simulink library "FAM_simple_lab_scale"  (R2023b)
settings: Solver=VariableStepAuto  StartTime=0.0  StopTime=10.0  RelTol=1e-3
undefined symbols (not defined in the file): FAM_elasticity, FAM_unstretched_length, FAM_unstretched_radius, FAM_wall_thickness, fiber_angle_alpha
settings Model: Creator=Carson  LastModifiedBy=Carson

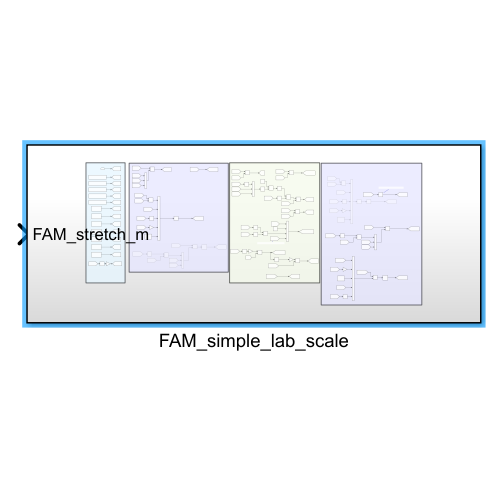
[thumbnail: Simulink's stored preview of the top-level diagram]
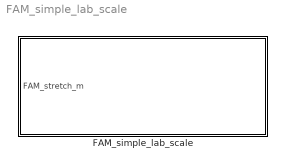
== system FAM_simple_lab_scale ==
  FAM_simple_lab_scale : Subsystem

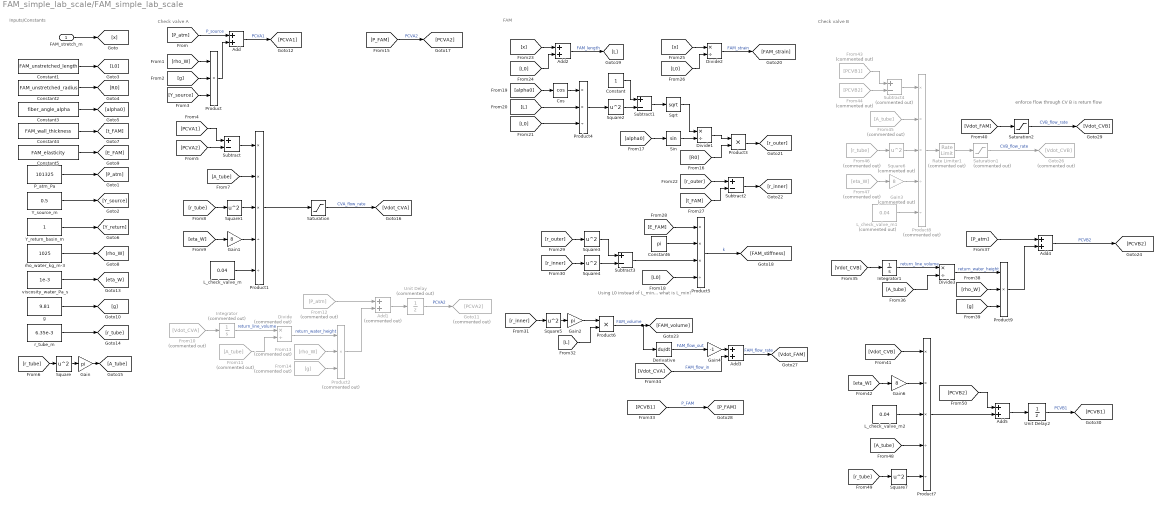
== system FAM_simple_lab_scale/FAM_simple_lab_scale ==
  note: enforce flow through CV B is return flow
  note: Check valve A
  note: Inputs/Constants
  note: FAM
  note: Using L0 instead of L_min... what is L_min?
  note: Check valve B
  FAM_stretch_m : Inport  Unit=m
  Add{,2..5} (5 alike) : Sum
  Add1 : Sum  Commented=on
  Constant : Constant
  Constant1 : Constant  Value=FAM_unstretched_length
  Constant2 : Constant  Value=FAM_unstretched_radius
  Constant3 : Constant  Value=fiber_angle_alpha
  Constant4 : Constant  Value=FAM_wall_thickness
  Constant5 : Constant  Value=FAM_elasticity
  Constant6 : Constant  Value=pi
  Cos : Trigonometry  Operator=cos
  Derivative : Derivative
  Divide : Product  Commented=on  Inputs=*/
  Divide1 : Product  Inputs=*/
  Divide2 : Product  Inputs=*/
  Divide3 : Product  Inputs=*/
  From10 : From  Commented=on  GotoTag=Vdot_CVA
  From11 : From  Commented=on  GotoTag=A_tube
  From12 : From  Commented=on  GotoTag=P_atm
  From13 : From  Commented=on  GotoTag=rho_W
  From14 : From  Commented=on  GotoTag=g
  From43 : From  Commented=on  GotoTag=PCVB1
  From44 : From  Commented=on  GotoTag=PCVB2
  From45 : From  Commented=on  GotoTag=A_tube
  From46 : From  Commented=on  GotoTag=r_tube
  From47 : From  Commented=on  GotoTag=eta_W
  Gain : Gain  Gain=pi
  Gain1 : Gain  Gain=8
  Gain2 : Gain  Gain=pi
  Gain3 : Gain  Commented=on  Gain=8
  Gain4 : Gain  Gain=-1
  Gain6 : Gain  Gain=8
  Goto11 : Goto  Commented=on  GotoTag=PCVA2
  Goto26 : Goto  Commented=on  GotoTag=Vdot_CVB
  Integrator : Integrator  Commented=on
  Integrator1 : Integrator
  L_check_valve_m : Constant  Value=0.04
  L_check_valve_m1 : Constant  Commented=on  Value=0.04
  L_check_valve_m2 : Constant  Value=0.04
  P_atm_Pa : Constant  Value=101325
  Product : Product  Inputs=***
  Product1 : Product  Inputs=***//
  Product2 : Product  Commented=on  Inputs=***
  Product3 : Product
  Product4 : Product  Inputs=**/
  Product5 : Product  Inputs=***/
  Product6 : Product
  Product7 : Product  Inputs=***//
  Product8 : Product  Commented=on  Inputs=***//
  Product9 : Product  Inputs=***
  Rate Limiter1 : RateLimiter  Commented=on  RisingSlewLimit=0.01  FallingSlewLimit=-0.01  SampleTimeMode=inherited
  Saturation : Saturate  UpperLimit=1e-4  LowerLimit=0
  Saturation1 : Saturate  Commented=on  UpperLimit=inf  LowerLimit=0
  Saturation2 : Saturate  UpperLimit=inf  LowerLimit=0  ZeroCross=off
  Sin : Trigonometry
  Sqrt : Sqrt
  Square{,1..5,7} (7 alike) : Math  Operator=square
  Square6 : Math  Commented=on  Operator=square
  Subtract{,1..3} (4 alike) : Sum  Inputs=+-
  Subtract4 : Sum  Commented=on  Inputs=+-
  Unit Delay : UnitDelay  Commented=on  InitialCondition=101325  SampleTime=-1  HasFrameUpgradeWarning=on
  Unit Delay2 : UnitDelay  InitialCondition=101325  SampleTime=-1  HasFrameUpgradeWarning=on
  Y_return_basin_m : Constant
  Y_source_m : Constant  Value=0.5
  g : Constant  Value=9.81
  r_tube_m : Constant  Value=6.35e-3
  rho_water_kg_m-3 : Constant  Value=1025
  viscosity_water_Pa_s : Constant  Value=1e-3
  wires:
  Y_return_basin_m/1 -> [Y_return]
  FAM_stretch_m/1 -> [x]
  Y_source_m/1 -> [Y_source]
  Constant4/1 -> [t_FAM]
  P_atm_Pa/1 -> [P_atm]
  rho_water_kg_m-3/1 -> [rho_W]
  Constant2/1 -> [R0]
  Constant5/1 -> [E_FAM]
  Constant1/1 -> [L0]
  Constant3/1 -> [alpha0]
  g/1 -> [g]
  [P_atm] -> Add/1  "P_source"
  Product/1 -> Add/2
  [rho_W] -> Product/1
  [g] -> Product/2
  [Y_source] -> Product/3
  Add/1 -> [PCVA1]  "PCVA1"
  viscosity_water_Pa_s/1 -> [eta_W]
  r_tube_m/1 -> [r_tube]
  [r_tube] -> Square/1
  Square/1 -> Gain/1
  Gain/1 -> [A_tube]
  Unit Delay/1 -> Goto11/1  "PCVA2"
  [PCVA1] -> Subtract/1
  [PCVA2] -> Subtract/2
  Subtract/1 -> Product1/1
  [A_tube] -> Product1/2
  [r_tube] -> Square1/1
  Square1/1 -> Product1/3
  [eta_W] -> Gain1/1
  Gain1/1 -> Product1/4
  L_check_valve_m/1 -> Product1/5
  Saturation/1 -> [Vdot_CVA]  "CVA_flow_rate"
  From10/1 -> Integrator/1
  Integrator/1 -> Divide/1  "return_line_volume"
  From11/1 -> Divide/2
  Divide/1 -> Product2/1  "return_water_height"
  Product2/1 -> Add1/2
  Add1/1 -> Unit Delay/1
  From12/1 -> Add1/1
  From13/1 -> Product2/2
  From14/1 -> Product2/3
  Product1/1 -> Saturation/1
  [P_FAM] -> [PCVA2]  "PCVA2"
  [x] -> Divide2/1
  [L0] -> Divide2/2
  Divide2/1 -> [FAM_strain]  "FAM_strain"
  Add2/1 -> [L]  "FAM_length"
  [L0] -> Add2/2
  [x] -> Add2/1
  [r_inner] -> Square4/1
  [alpha0] -> Sin/1
  Sin/1 -> Divide1/2
  Square4/1 -> Subtract3/2
  Product4/1 -> Square2/1
  Square3/1 -> Subtract3/1
  [L] -> Product4/2
  Sqrt/1 -> Divide1/1
  [L0] -> Product4/3
  Subtract2/1 -> [r_inner]
  [r_outer] -> Subtract2/1
  Divide1/1 -> Product3/1
  Constant6/1 -> Product5/2
  Square2/1 -> Subtract1/2
  [r_outer] -> Square3/1
  [L0] -> Product5/4
  Constant/1 -> Subtract1/1
  Subtract1/1 -> Sqrt/1
  Cos/1 -> Product4/1
  Product3/1 -> [r_outer]
  Subtract3/1 -> Product5/3
  [alpha0] -> Cos/1
  [t_FAM] -> Subtract2/2
  Product5/1 -> [FAM_stiffness]  "k"
  [R0] -> Product3/2
  [E_FAM] -> Product5/1
  Square5/1 -> Gain2/1
  [r_inner] -> Square5/1
  Gain2/1 -> Product6/1
  [L] -> Product6/2
  Product6/1 -> [FAM_volume], Derivative/1  "FAM_volume"
  Rate Limiter1/1 -> Saturation1/1
  Product8/1 -> Rate Limiter1/1
  [g] -> Product9/3
  [rho_W] -> Product9/2
  [P_atm] -> Add4/1
  Product9/1 -> Add4/2
  Divide3/1 -> Product9/1  "return_water_height"
  [A_tube] -> Divide3/2
  Integrator1/1 -> Divide3/1  "return_line_volume"
  [Vdot_CVB] -> Integrator1/1
  Saturation1/1 -> Goto26/1  "CVB_flow_rate"
  L_check_valve_m1/1 -> Product8/5
  Gain3/1 -> Product8/4
  From47/1 -> Gain3/1
  Square6/1 -> Product8/3
  From46/1 -> Square6/1
  From45/1 -> Product8/2
  Subtract4/1 -> Product8/1
  From44/1 -> Subtract4/2
  From43/1 -> Subtract4/1
  Add4/1 -> [PCVB2]  "PCVB2"
  Derivative/1 -> Gain4/1  "FAM_flow_out"
  [Vdot_CVA] -> Add3/2  "FAM_flow_in"
  Gain4/1 -> Add3/1
  Add3/1 -> [Vdot_FAM]  "FAM_flow_rate"
  Saturation2/1 -> [Vdot_CVB]  "CVB_flow_rate"
  [Vdot_CVB] -> Product7/1
  [eta_W] -> Gain6/1
  Gain6/1 -> Product7/2
  L_check_valve_m2/1 -> Product7/3
  [A_tube] -> Product7/4
  [r_tube] -> Square7/1
  Square7/1 -> Product7/5
  Product7/1 -> Add5/2
  [PCVB2] -> Add5/1
  Add5/1 -> Unit Delay2/1
  [PCVB1] -> [P_FAM]  "P_FAM"
  [Vdot_FAM] -> Saturation2/1
  Unit Delay2/1 -> [PCVB1]  "PCVB1"
